simulink model "HardwareControlNull"  (R2015a)
settings: configuration reference "SIMULATION_CONFIGURATION" (kept outside this file)
settings Model: Creator=moritz  LastModifiedBy=moritz
settings ConfigSetRef: SourceLocation=Base Workspace

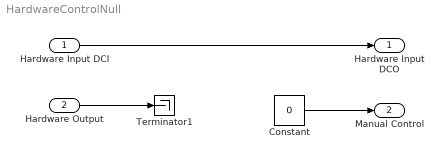
== system HardwareControlNull ==
  Hardware Input DCI : Inport  OutDataTypeStr=Bus: HARDWARE_IO_INPUT_BUS  BusOutputAsStruct=on
  Hardware Output : Inport  Port=2  OutDataTypeStr=Bus: HARDWARE_IO_OUTPUT_BUS
  Constant : Constant  Value=0  OutDataTypeStr=boolean
  Terminator1 : Terminator
  Hardware Input DCO : Outport  OutDataTypeStr=Bus: HARDWARE_IO_INPUT_BUS  BusOutputAsStruct=on
  Manual Control : Outport  Port=2
  wires:
  Constant/1 -> Manual Control/1
  Hardware Input DCI/1 -> Hardware Input DCO/1
  Hardware Output/1 -> Terminator1/1
